simulink model "udp_interface"  (R2015a)
settings: Solver=FixedStepDiscrete  SolverMode=SingleTasking  StartTime=0.0  StopTime=inf  FixedStep=0.004  RelTol=1e-3
undefined symbols (not defined in the file): dcar1_lib, packUDP, Standard_Devices, UDP_Protocol
libraries: sldrtlib x2, simulink x1
settings Model: sg_rtwmakecfg_data=_sg_IO821_  CovModelRefEnable=off  Creator=lab1  LastModifiedBy=VadBut
settings SolverCC: EnableConcurrentExecution=on
settings DataIOCC: SaveFormat=StructureWithTime  InspectSignalLogs=on
settings OptimizationCC: BlockReduction=off  OptimizeBlockIOStorage=off  BufferReuse=off  GlobalBufferReuse=off  ExpressionFolding=off  LocalBlockOutputs=off
settings DebuggingCC: ReadBeforeWriteMsg=DisableAll  WriteAfterWriteMsg=DisableAll  WriteAfterReadMsg=DisableAll  UnconnectedInputMsg=none  UnconnectedOutputMsg=none  UnconnectedLineMsg=none  UniqueDataStoreMsg=error
settings HardwareCC: ProdIntDivRoundTo=Zero  ProdEndianess=LittleEndian  ProdLongLongMode=on  ProdHWDeviceType=Generic->32-bit x86 compatible
settings RTWCC: SystemTargetFile=slrt.tlc  TemplateMakefile=slrt_default_tmf  Description=Simulink Real-Time  GenerateReport=on  LaunchReport=on  CodeExecutionProfiling=on  CodeProfilingInstrumentation=on  RTWCompilerOptimization=on
settings SimulinkRealTimeCC: GeneratePreprocessorConditionals=Disable all  xPCisModelTimeout=off  xPCModelTimeoutSecs=20

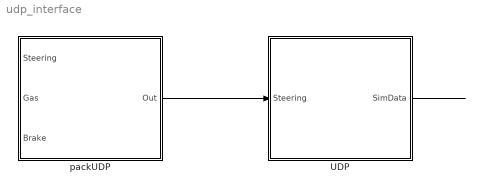
== system udp_interface ==
  UDP : Subsystem
  packUDP : Subsystem  AncestorBlock=dcar1_lib/packUDP
  wires:
  packUDP/1(Out) -> UDP/1(Steering)
  UDP/1(SimData) -> ?
  ? -> packUDP/1(Steering)
  ? -> packUDP/2(Gas)
  ? -> packUDP/3(Brake)

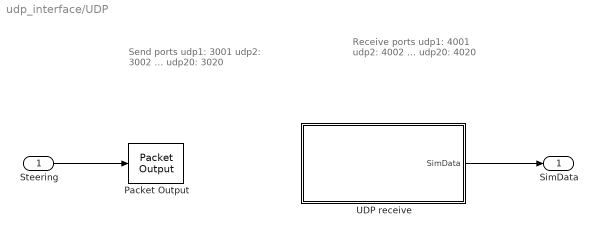
== system udp_interface/UDP ==
  note: Send ports
      | udp1: 3001
      | udp2: 3002
      | ...
      | udp20: 3020
  note: Receive ports
      | udp1: 4001
      | udp2: 4002
      | ...
      | udp20: 4020
  Steering : Inport
  Packet Output : sldrtlib/Packet Output  SampleTime=0.004  MaxMissedTicks=inf  ShowMissedTicks=off  YieldWhenWaiting=off  DrvName=Standard_Devices/UDP_Protocol  DrvAddress=-1  DrvOptions=[3232238661 3001]  PacketSize=18  DataTypes={'18*uint8'}  ShowReady=off  ShowError=off  PacketID=1  ByteOrder=1  InitialValue=[]  FinalValue=[]
      settings: AttributesFormatString=Standard Devices\nUDP Protocol [-1.000000e+00h]
  UDP receive : Subsystem
  SimData : Outport
  wires:
  UDP receive/1(SimData) -> SimData/1
  Steering/1 -> Packet Output/1

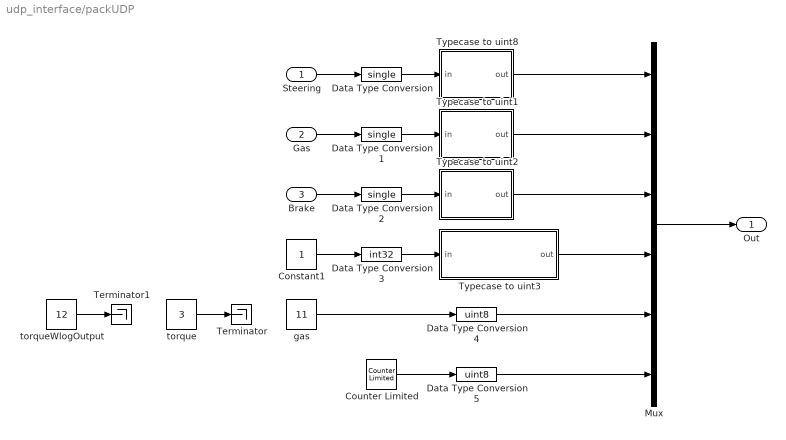
== system udp_interface/packUDP ==
  Steering : Inport
  Gas : Inport  Port=2
  Brake : Inport  Port=3
  Constant1 : Constant
  Counter Limited : simulink/Sources/Counter Limited  uplimit=255  tsamp=-1
  Data Type Conversion : DataTypeConversion  OutDataTypeStr=single
  Data Type Conversion1 : DataTypeConversion  OutDataTypeStr=single
  Data Type Conversion2 : DataTypeConversion  OutDataTypeStr=single
  Data Type Conversion3 : DataTypeConversion  OutDataTypeStr=int32
  Data Type Conversion4 : DataTypeConversion  OutDataTypeStr=uint8
  Data Type Conversion5 : DataTypeConversion  OutDataTypeStr=uint8
  Mux : Mux  Inputs=6
  Terminator : Terminator
  Terminator1 : Terminator
  Typecase to uint1 : MATLAB Function  TreatAsAtomicUnit=on
  Typecase to uint2 : MATLAB Function  TreatAsAtomicUnit=on
  Typecase to uint3 : MATLAB Function  TreatAsAtomicUnit=on
  Typecase to uint8 : MATLAB Function  TreatAsAtomicUnit=on
  gas : Constant  Value=11
  torque : Constant  Value=3
  torqueWlogOutput : Constant  Value=12
  Out : Outport
  wires:
  Counter Limited/1 -> Data Type Conversion5/1
  Data Type Conversion5/1 -> Mux/6
  gas/1 -> Data Type Conversion4/1
  Data Type Conversion4/1 -> Mux/5
  Data Type Conversion3/1 -> Typecase to uint3/1(in)
  Data Type Conversion2/1 -> Typecase to uint2/1(in)
  Data Type Conversion1/1 -> Typecase to uint1/1(in)
  Data Type Conversion/1 -> Typecase to uint8/1(in)
  Typecase to uint3/1(out) -> Mux/4
  Brake/1 -> Data Type Conversion2/1
  Typecase to uint2/1(out) -> Mux/3
  Constant1/1 -> Data Type Conversion3/1
  Typecase to uint1/1(out) -> Mux/2
  Gas/1 -> Data Type Conversion1/1
  Steering/1 -> Data Type Conversion/1
  Typecase to uint8/1(out) -> Mux/1
  Mux/1 -> Out/1
  torque/1 -> Terminator/1
  torqueWlogOutput/1 -> Terminator1/1

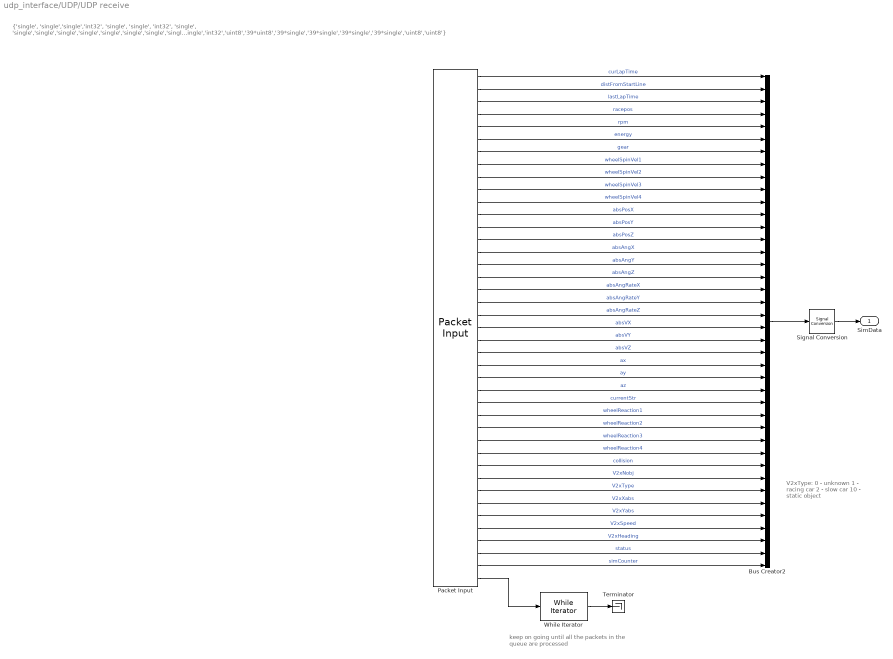
== system udp_interface/UDP/UDP receive ==
  note: {'single', 'single','single','int32', 'single', 'single', 'int32', 'single', 'single','single','single','single','single','single','single','single','single','single','single','single','single','single','single','single','single','single','single','single','single','single','single','int32','uint8','39*uint8','39*single','39*single','39*single','39*single','uint8','uint8'}
  note: keep on going until all the packets in the queue are processed
  note: V2xType:
      | 0 - unknown
      | 1 - racing car
      | 2 - slow car
      | 10 - static object
  Bus Creator2 : BusCreator  Inputs=40
  Packet Input : sldrtlib/Packet Input  SampleTime=-1  MaxMissedTicks=inf  ShowMissedTicks=off  YieldWhenWaiting=off  DrvName=Standard_Devices/UDP_Protocol  DrvAddress=4001  DrvOptions=[0 -1]  PacketSize=794  DataTypes={'single', 'single','single','int32', 'single', 'single', 'int32', 'single', 'single','single','single','single','single','single','single','single','single','single','single','single','single','single','single','single','single','single','single','single','single','single','single','int32','uint8','39*uint8','39*single','39*single','39*single','39*single','uint8','uint8'}  ShowReady=on  ShowError=off  PacketID=1  ByteOrder=1  ShowTimestamp=off
      settings: AttributesFormatString=Standard Devices\nUDP Protocol [FA1h]
  Signal Conversion : SignalConversion
  Terminator : Terminator
  While Iterator : WhileIterator  MaxIters=-1  WhileBlockType=do-while  ShowIterationPort=on  OutputDataType=int8
  SimData : Outport
  wires:
  Signal Conversion/1 -> SimData/1
  While Iterator/1 -> Terminator/1
  Packet Input/1 -> Bus Creator2/1  "curLapTime"
  Packet Input/2 -> Bus Creator2/2  "distFromStartLine"
  Packet Input/3 -> Bus Creator2/3  "lastLapTime"
  Packet Input/4 -> Bus Creator2/4  "racepos"
  Packet Input/6 -> Bus Creator2/6  "energy"
  Packet Input/9 -> Bus Creator2/9  "wheelSpinVel2"
  Packet Input/12 -> Bus Creator2/12  "absPosX"
  Packet Input/18 -> Bus Creator2/18  "absAngRateX"
  Packet Input/21 -> Bus Creator2/21  "absVX"
  Packet Input/24 -> Bus Creator2/24  "ax"
  Packet Input/15 -> Bus Creator2/15  "absAngX"
  Packet Input/30 -> Bus Creator2/30  "wheelReaction3"
  Packet Input/27 -> Bus Creator2/27  "currentStr"
  Packet Input/26 -> Bus Creator2/26  "az"
  Packet Input/29 -> Bus Creator2/29  "wheelReaction2"
  Packet Input/11 -> Bus Creator2/11  "wheelSpinVel4"
  Packet Input/5 -> Bus Creator2/5  "rpm"
  Packet Input/8 -> Bus Creator2/8  "wheelSpinVel1"
  Packet Input/17 -> Bus Creator2/17  "absAngZ"
  Packet Input/14 -> Bus Creator2/14  "absPosZ"
  Packet Input/20 -> Bus Creator2/20  "absAngRateZ"
  Packet Input/23 -> Bus Creator2/23  "absVZ"
  Packet Input/31 -> Bus Creator2/31  "wheelReaction4"
  Packet Input/22 -> Bus Creator2/22  "absVY"
  Packet Input/25 -> Bus Creator2/25  "ay"
  Packet Input/28 -> Bus Creator2/28  "wheelReaction1"
  Packet Input/13 -> Bus Creator2/13  "absPosY"
  Packet Input/16 -> Bus Creator2/16  "absAngY"
  Packet Input/19 -> Bus Creator2/19  "absAngRateY"
  Packet Input/7 -> Bus Creator2/7  "gear"
  Packet Input/10 -> Bus Creator2/10  "wheelSpinVel3"
  Bus Creator2/1 -> Signal Conversion/1
  Packet Input/33 -> Bus Creator2/33  "V2xNobj"
  Packet Input/34 -> Bus Creator2/34  "V2xType"
  Packet Input/35 -> Bus Creator2/35  "V2xXabs"
  Packet Input/39 -> Bus Creator2/39  "status"
  Packet Input/38 -> Bus Creator2/38  "V2xHeading"
  Packet Input/36 -> Bus Creator2/36  "V2xYabs"
  Packet Input/37 -> Bus Creator2/37  "V2xSpeed"
  Packet Input/40 -> Bus Creator2/40  "simCounter"
  Packet Input/32 -> Bus Creator2/32  "collision"
  Packet Input/41 -> While Iterator/1

== matlab function udp_interface/packUDP/Typecase to uint3 ==
  data: in input int32 size=[1 1]; out output uint8 size=[1 4]
function out = cast_int32_to_uint8(in)

out = typecast(in,'uint8');

== matlab function udp_interface/packUDP/Typecase to uint8 ==
  data: in input single size=[1 1]; out output uint8 size=[1 4]
function out = cast_uint8(in)

out = typecast(in,'uint8');

== matlab function udp_interface/packUDP/Typecase to uint1 ==
  data: in input single size=[1 1]; out output uint8 size=[1 4]
function out = cast_uint8(in)

out = typecast(in,'uint8');

== matlab function udp_interface/packUDP/Typecase to uint2 ==
  data: in input single size=[1 1]; out output uint8 size=[1 4]
function out = cast_uint8(in)

out = typecast(in,'uint8');
